simulink model "quantizer_uniform"  (Simulink 7.9)
settings: Solver=FixedStepDiscrete  SolverMode=SingleTasking  StartTime=0.0  StopTime=1  FixedStep=1/10000  RelTol=1e-3  AbsTol=1e-6
values from neighbouring files (symbols this model uses):
  k = 1/4.902/(sqrt(10^(atenuation_dB/10)))    [quant_non_uniform.m]    (also in quant_uniform.m; speech_quant_non_uniform.m = sqrt(10^(atenuation_dB/10)); speech_quant_uniform.m = sqrt(10^(atenuation_dB/10)))
libraries: dspquant2 x1
settings Model: Creator=amoura  LastModifiedBy=amoura_2
settings DataIOCC: LimitDataPoints=off
settings OptimizationCC: BlockReduction=off  BooleanDataType=off  InitFltsAndDblsToZero=on
settings DebuggingCC: SaveWithParameterizedLinksMsg=none  SignalResolutionControl=TryResolveAllWithWarning  SolverPrmCheckMsg=none  MultiTaskDSMMsg=warning  MultiTaskCondExecSysMsg=none  FcnCallInpInsideContextMsg=Use local settings  StrictBusMsg=None
settings HardwareCC: TargetUnknown=on
settings RTWCC: TemplateMakefile=grt_unix.tmf  IncludeERTFirstTime=on
settings GRTTargetCC: TargetFcnLib=ansi_tfl_tmw.mat  ModelReferenceCompliant=off  CombineOutputUpdateFcns=off  MatFileLogging=off  GRTInterface=on

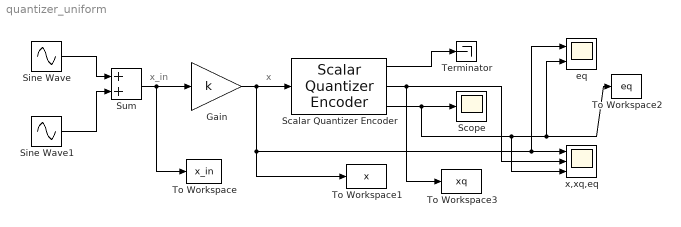
== system quantizer_uniform ==
  note: x
  note: x_in
  Gain : Gain  Gain=k  SaturateOnIntegerOverflow=on  OutDataTypeStr=Inherit: Same as input  ParamDataTypeStr=Inherit: Same as input
  Scalar Quantizer Encoder : dspquant2/Scalar Quantizer Encoder  paramSrc=Specify via dialog  partType=Bounded  BBoundary=boundary  UBoundary=[2:9]  SearchMethod=Linear  tieBreakRule=Choose the lower index  outQU=on  outQError=on  codebook=codebook  outStatus=off  invalidin=Clip  idtype=int32  roundingMode=Floor  overflowMode=off
  Scope : Scope
      settings: TickLabels=on
  Sine Wave : Sin  Amplitude=3  Frequency=2*pi*20  SampleTime=0
  Sine Wave1 : Sin  Amplitude=2  Frequency=2*pi*120  SampleTime=0
  Sum : Sum  SaturateOnIntegerOverflow=on  InputSameDT=on  OutDataTypeStr=Inherit: Same as first input
  Terminator : Terminator
  To Workspace : ToWorkspace  VariableName=x_in  SampleTime=-1
  To Workspace1 : ToWorkspace  VariableName=x  SampleTime=-1
  To Workspace2 : ToWorkspace  VariableName=eq  SampleTime=-1
  To Workspace3 : ToWorkspace  VariableName=xq  SampleTime=-1
  eq : Scope  NumInputPorts=2
      settings: TickLabels=on  YMin=-1~-1  YMax=1~1
  x,xq,eq : Scope  NumInputPorts=3
      settings: TickLabels=on  YMin=-1.5~-1.5~-1.5  YMax=1.5~1.5~1.5
  wires:
  Sum/1 -> To Workspace/1, Gain/1
  Scalar Quantizer Encoder/2 -> To Workspace3/1, x,xq,eq/2
  Gain/1 -> To Workspace1/1, x,xq,eq/1, eq/1, Scalar Quantizer Encoder/1
  Scalar Quantizer Encoder/3 -> Scope/1, To Workspace2/1, eq/2, x,xq,eq/3
  Scalar Quantizer Encoder/1 -> Terminator/1
  Sine Wave1/1 -> Sum/2
  Sine Wave/1 -> Sum/1
